simulink model "Project3_Part2_sim"  (R2018a)
(part 3 of 4)

CFG = [t1033+t1034+t1035+t1036+t1037+t1038+t1040+t1041+thDot1.*3.0-t433.*(t2.*3.99066170156947e-3+t251)+t202.*(t213+t241+t245+t250+t259+t271+t272+t276+t277+t281+t283+t287+t291+t292+t293+t294+t295+t296+t297+t298+t299+t300+t301+t302+t303+t304+t305+t306+t307+t308+t402+t405+t406+t407+t408+t442+t446-t2.*t14.*1.25890039900759e-2-t62.*t133.*1.139953928995173-t14.*t253.*7.377352061241174e1-t404.*thDot1.*4.38483060303202-t131.*(t183+t184+t186+t222-t8.*t27.*t109).*1.994855465224146-t2.*t12.*t14.*9.450145625450081e-1-t2.*t12.*t84.*9.450145625450081e-1-t2.*t12.*t86.*9.450145625450081e-1-t2.*t27.*t266.*4.38483060303202-t2.*t3.*t7.*t14.*1.865719029901695e-3-t2.*t3.*t7.*t84.*1.865719029901695e-3-t2.*t3.*t7.*t86.*1.865719029901695e-3-t2.*t3.*t7.*t87.*1.865719029901695e-3-t2.*t14.*t89.*t90.*1.547905453732908-t2.*t84.*t89.*t90.*1.547905453732908-t2.*t86.*t89.*t90.*1.547905453732908-t12.*t27.*t113.*thDot4.*1.900321864457165e1-t2.*t12.*thDot2.*thDot3.*1.890029125090016-t8.*t182.*thDot1.*thDot2.*3.812773007925995e1-t2.*t3.*t7.*thDot2.*thDot3.*3.73143805980339e-3-t4.*t7.*t8.*thDot1.*thDot4.*3.73143805980339e-3-t3.*t8.*t12.*thDot1.*thDot2.*3.73143805980339e-3-t3.*t8.*t12.*thDot1.*thDot3.*3.73143805980339e-3-t2.*t89.*t90.*thDot2.*thDot3.*3.095810907465815)+t33.*(t836+t33.*(t827+t828-t2.*t8.*t92.*2.36837910197578e-2)-t109.*t831)-t742.*(t213+t241+t245+t250+t259+t271+t272+t276+t277+t281+t283+t287+t291+t292+t293+t294+t295+t296+t297+t298+t299+t300+t301+t302+t303+t304+t305+t306+t307+t308+t507+t508+t509+t510-t2.*t14.*4.310799465649219e-3-t62.*t133.*1.139953928995173-t131.*t314.*1.994855465224146-t2.*t12.*t14.*9.450145625450081e-1-t2.*t12.*t84.*9.450145625450081e-1-t2.*t12.*t86.*9.450145625450081e-1-t2.*t3.*t7.*t14.*1.865719029901695e-3-t2.*t3.*t7.*t84.*1.865719029901695e-3-t2.*t3.*t7.*t86.*1.865719029901695e-3-t2.*t3.*t7.*t87.*1.865719029901695e-3-t2.*t14.*t89.*t90.*1.547905453732908-t2.*t84.*t89.*t90.*1.547905453732908-t2.*t86.*t89.*t90.*1.547905453732908-t12.*t27.*t113.*thDot4.*1.900321864457165e1-t2.*t12.*thDot2.*thDot3.*1.890029125090016-t2.*t3.*t7.*thDot2.*thDot3.*3.73143805980339e-3-t4.*t7.*t8.*thDot1.*thDot4.*3.73143805980339e-3-t3.*t8.*t12.*thDot1.*thDot2.*3.73143805980339e-3-t3.*t8.*t12.*thDot1.*thDot3.*3.73143805980339e-3-t2.*t89.*t90.*thDot2.*thDot3.*3.095810907465815)+t959.*(t340+t342+t347+t348+t349+t363+t364+t365+t366+t367+t368+t369+t370+t371+t372+t373+t377+t378+t379+t380+t563+t564+t565+t566+t567+t568+t569+t570+t571+t572+t573-t71.*t123.*1.139953928995173-t145.*t152.*1.139953928995173-t104.*t221.*1.994855465224146-t36.*t339.*1.994855465224146-t36.*t352.*1.139953928995173-t131.*t394.*1.994855465224146-t8.*t14.*t85.*8.455164471901305e-1-t8.*t84.*t85.*8.455164471901305e-1-t8.*t14.*t85.*t88.*2.191879307959464e-1-t8.*t84.*t85.*t88.*2.191879307959464e-1-t8.*t85.*t86.*t88.*2.191879307959464e-1-t2.*t4.*t7.*thDot1.*thDot4.*3.73143805980339e-3-t2.*t3.*t12.*thDot1.*thDot2.*3.73143805980339e-3-t2.*t3.*t12.*thDot1.*thDot3.*3.73143805980339e-3-t4.*t8.*t12.*thDot2.*thDot4.*3.73143805980339e-3-t4.*t8.*t12.*thDot3.*thDot4.*3.73143805980339e-3-t3.*t8.*t91.*thDot1.*thDot4.*3.73143805980339e-3-t3.*t8.*t92.*thDot1.*thDot4.*3.73143805980339e-3-t8.*t85.*t88.*thDot2.*thDot3.*4.383758615918928e-1)+t230.*(t340+t342+t347+t348+t349+t363+t364+t365+t366+t367+t368+t369+t370+t371+t372+t373+t374+t375+t376+t377+t378+t379+t380+t381+t382+t383+t384+t385+t386+t391+t398+t399+t400+t401-t434-t435-t436+t485-t486-t487-t488-t489-t490-t491-t492-t493-t494-t495-t496-t497-t498-t499-t500-t501-t502-t503-t504)+t172.*t438-t71.*t553-t226.*t433-t167.*t506-t140.*t597-t179.*t676-t134.*t730-t108.*t877-t107.*t890-t113.*t887-t290.*t711-t62.*t955-t314.*t733-t114.*t964-t397.*t713+t438.*t746+t553.*t901-t941.*(t340+t342+t347+t348+t349+t363+t364+t365+t366+t367+t368+t369+t370+t371+t372+t373+t374+t375+t376+t377+t378+t379+t380+t381+t382+t383+t384+t385+t398+t518+t519+t520-t71.*t123.*1.139953928995173-t33.*t211.*1.900321864457165e1-t145.*t152.*1.139953928995173-t104.*t221.*1.994855465224146-t36.*t339.*1.994855465224146-t36.*t352.*1.139953928995173-t109.*t344.*1.900321864457165e1-t131.*t394.*1.994855465224146-t8.*t14.*t85.*5.971038255043736-t8.*t84.*t85.*5.971038255043736-t8.*t14.*t85.*t88.*1.547905453732908-t8.*t84.*t85.*t88.*1.547905453732908-t8.*t85.*t86.*t88.*1.547905453732908-t12.*t27.*t179.*thDot4.*1.900321864457165e1-t2.*t4.*t7.*thDot1.*thDot4.*3.73143805980339e-3-t2.*t3.*t12.*thDot1.*thDot2.*3.73143805980339e-3-t2.*t3.*t12.*thDot1.*thDot3.*3.73143805980339e-3-t4.*t8.*t12.*thDot2.*thDot4.*3.73143805980339e-3-t4.*t8.*t12.*thDot3.*thDot4.*3.73143805980339e-3-t3.*t8.*t91.*thDot1.*thDot4.*3.73143805980339e-3-t3.*t8.*t92.*thDot1.*thDot4.*3.73143805980339e-3-t8.*t85.*t88.*thDot2.*thDot3.*3.095810907465815)-t7.*thDot4.*(1.0./1.0e1)-t64.*thDot6.*(1.0./2.0e1)-t506.*(t8.*3.99066170156947e-3-t201)+t683.*(t213+t241+t245+t250+t259+t464+t465+t466+t467+t468+t469+t470+t471+t472+t473+t474+t475+t476+t477+t478+t479+t480+t481+t482+t483+t484+t156.*(t21+t22+t23-t12.*thDot2.*thDot4-t12.*thDot3.*thDot4).*1.139953928995173-t2.*t14.*2.219760847427988e-4-t62.*t133.*1.139953928995173+t78.*(t183+t184+t185+t186-t36.*(t28+t32+t42-t2.*t12.*thDot4)+(thDot1-t7.*thDot4).*(t28+t32-t2.*t12.*thDot4)+t8.*t27.*(t34-thDot1)).*1.139953928995173-t2.*t12.*t14.*3.436486650567527e-1-t2.*t12.*t84.*3.436486650567527e-1-t2.*t12.*t86.*3.436486650567527e-1-t2.*t3.*t7.*t14.*6.784571152745185e-4-t2.*t3.*t7.*t84.*6.784571152745185e-4-t2.*t3.*t7.*t86.*6.784571152745185e-4-t2.*t3.*t7.*t87.*6.784571152745185e-4-t2.*t14.*t89.*t90.*7.970632707682899e-2-t2.*t84.*t89.*t90.*7.970632707682899e-2-t2.*t86.*t89.*t90.*7.970632707682899e-2-t2.*t12.*thDot2.*thDot3.*6.872973301135055e-1-t2.*t3.*t7.*thDot2.*thDot3.*1.356914230549037e-3-t4.*t7.*t8.*thDot1.*thDot4.*1.356914230549037e-3-t3.*t8.*t12.*thDot1.*thDot2.*1.356914230549037e-3-t3.*t8.*t12.*thDot1.*thDot3.*1.356914230549037e-3-t2.*t89.*t90.*thDot2.*thDot3.*1.59412654153658e-1)+t840.*(t213+t241+t245+t250+t259+t271+t276+t277+t283+t287+t292+t293+t297+t298+t299+t300+t301+t302+t303+t574+t575+t576+t577+t578+t579+t580+t581+t582+t583+t584+t585-t2.*t14.*6.104217881481557e-4-t62.*t133.*1.139953928995173-t131.*t314.*1.994855465224146-t2.*t12.*t14.*9.450145625450081e-1-t2.*t12.*t84.*9.450145625450081e-1-t2.*t12.*t86.*9.450145625450081e-1-t2.*t3.*t7.*t14.*1.865719029901695e-3-t2.*t3.*t7.*t84.*1.865719029901695e-3-t2.*t3.*t7.*t86.*1.865719029901695e-3-t2.*t3.*t7.*t87.*1.865719029901695e-3-t2.*t14.*t89.*t90.*2.191879307959464e-1-t2.*t84.*t89.*t90.*2.191879307959464e-1-t2.*t86.*t89.*t90.*2.191879307959464e-1-t2.*t12.*thDot2.*thDot3.*1.890029125090016-t2.*t3.*t7.*thDot2.*thDot3.*3.73143805980339e-3-t4.*t7.*t8.*thDot1.*thDot4.*3.73143805980339e-3-t3.*t8.*t12.*thDot1.*thDot2.*3.73143805980339e-3-t3.*t8.*t12.*thDot1.*thDot3.*3.73143805980339e-3-t2.*t89.*t90.*thDot2.*thDot3.*4.383758615918928e-1)+t253.*(t340+t342+t347+t348+t349+t363+t364+t365+t366+t367+t368+t369+t370+t371+t372+t373+t374+t375+t376+t377+t378+t379+t380+t381+t382+t383+t384+t385+t386+t391+t399+t400+t401+t429-t71.*t123.*1.139953928995173+t14.*t202.*7.377352061241174e1-t33.*t211.*1.900321864457165e1-t145.*t152.*1.139953928995173-t104.*t221.*1.994855465224146-t36.*t339.*1.994855465224146-t36.*t352.*1.139953928995173-t109.*t344.*1.900321864457165e1-t432.*thDot1.*3.812773007925995e1-t131.*(t124+t125+t126+t127-t2.*t27.*t109).*1.994855465224146+t164.*(t125+t127-t2.*t27.*t109).*1.900321864457165e1-t8.*t14.*t85.*7.153708691033507-t8.*t84.*t85.*7.153708691033507-t8.*t270.*thDot2.*3.812773007925995e1-t8.*t14.*t85.*t88.*1.547905453732908-t8.*t84.*t85.*t88.*1.547905453732908-t8.*t85.*t86.*t88.*1.547905453732908-t12.*t27.*t179.*thDot4.*1.900321864457165e1-t2.*t182.*thDot1.*thDot2.*3.812773007925995e1-t2.*t4.*t7.*thDot1.*thDot4.*3.73143805980339e-3-t2.*t3.*t12.*thDot1.*thDot2.*3.73143805980339e-3-t2.*t3.*t12.*thDot1.*thDot3.*3.73143805980339e-3-t4.*t8.*t12.*thDot2.*thDot4.*3.73143805980339e-3-t4.*t8.*t12.*thDot3.*thDot4.*3.73143805980339e-3-t3.*t8.*t91.*thDot1.*thDot4.*3.73143805980339e-3-t3.*t8.*t92.*thDot1.*thDot4.*3.73143805980339e-3-t8.*t85.*t88.*thDot2.*thDot3.*3.095810907465815)-t945.*(t340+t342+t347+t348+t349+t363+t364+t365+t366+t367+t368+t369+t370+t371+t372+t373+t374+t375+t376+t377+t378+t379+t380+t381+t382+t383+t384+t385+t386+t391+t398+t399+t400+t401+t485-t71.*t123.*1.139953928995173-t33.*t211.*1.900321864457165e1-t145.*t152.*1.139953928995173-t104.*t221.*1.994855465224146-t36.*t339.*1.994855465224146-t36.*t352.*1.139953928995173-t109.*t344.*1.900321864457165e1-t131.*t394.*1.994855465224146-t8.*t14.*t85.*7.153708691033507-t8.*t84.*t85.*7.153708691033507-t8.*t14.*t85.*t88.*1.547905453732908-t8.*t84.*t85.*t88.*1.547905453732908-t8.*t85.*t86.*t88.*1.547905453732908-t12.*t27.*t179.*thDot4.*1.900321864457165e1-t2.*t4.*t7.*thDot1.*thDot4.*3.73143805980339e-3-t2.*t3.*t12.*thDot1.*thDot2.*3.73143805980339e-3-t2.*t3.*t12.*thDot1.*thDot3.*3.73143805980339e-3-t4.*t8.*t12.*thDot2.*thDot4.*3.73143805980339e-3-t4.*t8.*t12.*thDot3.*thDot4.*3.73143805980339e-3-t3.*t8.*t91.*thDot1.*thDot4.*3.73143805980339e-3-t3.*t8.*t92.*thDot1.*thDot4.*3.73143805980339e-3-t8.*t85.*t88.*thDot2.*thDot3.*3.095810907465815)+t8.*t27.*t852+t2.*t27.*t967-t4.*t12.*thDot5.*(1.0./1.0e1)-t8.*t691.*thDot2-t2.*t904.*thDot2+t7.*t12.*t27.*t586.*thDot1.*9.31865436135962e-4+t7.*t12.*t27.*t587.*thDot1.*9.31865436135962e-4-t85.*t89.*t586.*thDot1.*thDot2.*1.778633004674423e-1-t85.*t89.*t587.*thDot1.*thDot2.*1.778633004674423e-1;t8.*(t1006+t1008+t1013+t1014+t1015+t1016+t1019+t1020+t1021+t1022+t1023+t1026+t1028+t1029+t1030+t1031+t1032+t683.*(t618+t619+t620+t621+t622+t623+t625+t626+t627+t628+t629+t630+t631+t632+t633+t634+t635+t636+t637+t638+t639+t640+t641+t642+t643+t644+t645+t646+t647+t648+t649+t650+t651+t652+t653+t654+t655+t656+t657+t658+t659+t660+t661+t856-t71.*t231.*1.139953928995173-t73.*t244.*1.139953928995173-t50.*t337.*1.139953928995173-t62.*t602.*1.139953928995173-t84.*t89.*t90.*3.436486650567527e-1-t86.*t89.*t90.*3.436486650567527e-1-t3.*t84.*t85.*t90.*6.784571152745185e-4-t3.*t84.*t88.*t89.*6.784571152745185e-4-t3.*t85.*t86.*t90.*6.784571152745185e-4-t3.*t85.*t87.*t90.*6.784571152745185e-4-t3.*t86.*t88.*t89.*6.784571152745185e-4-t3.*t87.*t88.*t89.*6.784571152745185e-4-t13.*t84.*t89.*t90.*1.199966622536514e-4-t13.*t86.*t89.*t90.*1.199966622536514e-4-t13.*t89.*t90.*t607.*1.199966622536514e-4-t89.*t90.*thDot2.*thDot3.*6.872973301135055e-1-t3.*t85.*t88.*thDot2.*thDot4.*4.530050512289873e-4-t3.*t85.*t88.*thDot3.*thDot4.*4.530050512289873e-4-t3.*t85.*t90.*thDot2.*thDot3.*1.356914230549037e-3-t4.*t85.*t88.*thDot2.*thDot4.*1.356914230549037e-3-t4.*t85.*t88.*thDot3.*thDot4.*1.356914230549037e-3-t3.*t88.*t89.*thDot2.*thDot3.*1.356914230549037e-3-t13.*t89.*t90.*thDot2.*thDot3.*2.399933245073028e-4-t4.*t11.*t89.*t90.*thDot2.*thDot4.*2.399933245073028e-4-t4.*t11.*t89.*t90.*thDot3.*thDot4.*2.399933245073028e-4-t4.*t13.*t85.*t90.*thDot4.*thDot5.*2.399933245073028e-4-t3.*t13.*t89.*t90.*thDot2.*thDot5.*2.399933245073028e-4-t3.*t13.*t89.*t90.*thDot3.*thDot5.*2.399933245073028e-4-t4.*t13.*t88.*t89.*thDot4.*thDot5.*2.399933245073028e-4+1.11715485041527e1)-t78.*t553-t164.*t676-t113.*t744-t175.*t737-t123.*t855-t397.*t601-t108.*t910-t394.*t680-t109.*t1025-t337.*t821+t597.*t889-t742.*t744+t746.*t826-t737.*t920-t880.*t1012+t8.*thDot2.*3.0+t691.*thDot1-t852.*thDot1-t62.*(t946+t949-t62.*t799)+t182.*(t340+t347+t348+t349+t363+t364+t365+t366+t367+t368+t369+t370+t371+t372+t373+t374+t375+t376+t377+t378+t379+t380+t381+t382+t383+t384+t385+t386+t391+t398+t399+t400+t401+t429-t434-t435-t436-t486-t487-t488-t489-t490-t491-t492-t493-t494-t495-t496-t497-t498-t499-t500-t501-t502-t503-t504+t723-t738-t739-t740)-t107.*(t608+t611+t612+t616+t617+t618+t619+t620+t621+t622+t623+t624+t625+t626+t627+t628+t629+t630+t631+t632+t633+t634+t635+t636+t637+t638+t639+t640+t641+t642+t643+t644+t645+t646+t647+t648+t649+t650+t651+t652+t653+t654+t655+t656+t657+t658+t659+t660+t661+t662+t841+t842+t843+t844-t71.*t231.*1.139953928995173-t73.*t244.*1.139953928995173-t104.*t275.*1.994855465224146-t50.*t337.*1.139953928995173-t140.*t314.*1.994855465224146-t62.*t602.*1.139953928995173-t84.*t604.*5.936309573135882e-4-t84.*t606.*5.936309573135882e-4-t86.*t604.*5.936309573135882e-4-t87.*t604.*5.936309573135882e-4-t86.*t606.*5.936309573135882e-4-t87.*t606.*5.936309573135882e-4-t84.*t89.*t90.*3.436486650567527e-1-t86.*t89.*t90.*3.436486650567527e-1-t604.*thDot2.*thDot3.*1.187261914627176e-3-t604.*thDot2.*thDot4.*1.187261914627176e-3-t604.*thDot3.*thDot4.*1.187261914627176e-3-t606.*thDot2.*thDot3.*1.187261914627176e-3-t3.*t84.*t85.*t90.*6.784571152745185e-4-t3.*t84.*t88.*t89.*6.784571152745185e-4-t3.*t85.*t86.*t90.*6.784571152745185e-4-t3.*t85.*t87.*t90.*6.784571152745185e-4-t3.*t86.*t88.*t89.*6.784571152745185e-4-t3.*t87.*t88.*t89.*6.784571152745185e-4-t13.*t84.*t89.*t90.*1.199966622536514e-4-t13.*t86.*t89.*t90.*1.199966622536514e-4-t13.*t89.*t90.*t607.*1.199966622536514e-4-t89.*t90.*thDot2.*thDot3.*6.872973301135055e-1-t3.*t85.*t88.*thDot2.*thDot4.*4.530050512289873e-4-t3.*t85.*t88.*thDot3.*thDot4.*4.530050512289873e-4-t3.*t85.*t90.*thDot2.*thDot3.*1.356914230549037e-3-t4.*t85.*t88.*thDot2.*thDot4.*1.356914230549037e-3-t4.*t85.*t88.*thDot3.*thDot4.*1.356914230549037e-3-t3.*t88.*t89.*thDot2.*thDot3.*1.356914230549037e-3-t13.*t89.*t90.*thDot2.*thDot3.*2.399933245073028e-4-t4.*t11.*t89.*t90.*thDot2.*thDot4.*2.399933245073028e-4-t4.*t11.*t89.*t90.*thDot3.*thDot4.*2.399933245073028e-4-t4.*t13.*t85.*t90.*thDot4.*thDot5.*2.399933245073028e-4-t3.*t13.*t89.*t90.*thDot2.*thDot5.*2.399933245073028e-4-t3.*t13.*t89.*t90.*thDot3.*thDot5.*2.399933245073028e-4-t4.*t13.*t88.*t89.*thDot4.*thDot5.*2.399933245073028e-4+3.072113206334932e1)-t167.*(t608+t609+t610+t611+t612+t613+t614+t615+t616+t617+t618+t619+t620+t621+t622+t623+t624+t625+t626+t627+t628+t629+t630+t631+t632+t633+t634+t635+t636+t637+t638+t639+t640+t641+t642+t643+t644+t645+t646+t647+t648+t649+t650+t651+t652+t653+t654+t655+t656+t657+t658+t659+t660+t661+t662+t748+t764+t770+t884+t885-t71.*t231.*1.139953928995173-t73.*t244.*1.139953928995173-t104.*t275.*1.994855465224146-t50.*t337.*1.139953928995173-t140.*t314.*1.994855465224146-t114.*t344.*1.900321864457165e1-t179.*t290.*1.900321864457165e1-t62.*t602.*1.139953928995173-t84.*t604.*5.936309573135882e-4-t84.*t606.*5.936309573135882e-4-t86.*t604.*5.936309573135882e-4-t87.*t604.*5.936309573135882e-4-t86.*t606.*5.936309573135882e-4-t87.*t606.*5.936309573135882e-4-t84.*t89.*t90.*3.436486650567527e-1-t86.*t89.*t90.*3.436486650567527e-1-t8.*t27.*t404.*4.38483060303202-t2.*t432.*thDot2.*3.812773007925995e1-t604.*thDot2.*thDot3.*1.187261914627176e-3-t604.*thDot2.*thDot4.*1.187261914627176e-3-t604.*thDot3.*thDot4.*1.187261914627176e-3-t606.*thDot2.*thDot3.*1.187261914627176e-3-t3.*t84.*t85.*t90.*6.784571152745185e-4-t3.*t84.*t88.*t89.*6.784571152745185e-4-t3.*t85.*t86.*t90.*6.784571152745185e-4-t3.*t85.*t87.*t90.*6.784571152745185e-4-t3.*t86.*t88.*t89.*6.784571152745185e-4-t3.*t87.*t88.*t89.*6.784571152745185e-4-t13.*t84.*t89.*t90.*1.199966622536514e-4-t13.*t86.*t89.*t90.*1.199966622536514e-4-t13.*t89.*t90.*t607.*1.199966622536514e-4-t2.*t27.*t172.*thDot1.*4.38483060303202-t89.*t90.*thDot2.*thDot3.*6.872973301135055e-1-t8.*t226.*thDot1.*thDot2.*3.812773007925995e1-t3.*t85.*t88.*thDot2.*thDot4.*4.530050512289873e-4-t3.*t85.*t88.*thDot3.*thDot4.*4.530050512289873e-4-t3.*t85.*t90.*thDot2.*thDot3.*1.356914230549037e-3-t4.*t85.*t88.*thDot2.*thDot4.*1.356914230549037e-3-t4.*t85.*t88.*thDot3.*thDot4.*1.356914230549037e-3-t3.*t88.*t89.*thDot2.*thDot3.*1.356914230549037e-3-t13.*t89.*t90.*thDot2.*thDot3.*2.399933245073028e-4-t4.*t11.*t89.*t90.*thDot2.*thDot4.*2.399933245073028e-4-t4.*t11.*t89.*t90.*thDot3.*thDot4.*2.399933245073028e-4-t4.*t13.*t85.*t90.*thDot4.*thDot5.*2.399933245073028e-4-t3.*t13.*t89.*t90.*thDot2.*thDot5.*2.399933245073028e-4-t3.*t13.*t89.*t90.*thDot3.*thDot5.*2.399933245073028e-4-t4.*t13.*t88.*t89.*thDot4.*thDot5.*2.399933245073028e-4+6.335757694666128e2)-t2.*t12.*thDot4.*(1.0./1.0e1)-t8.*t27.*t595.*thDot1-t2.*t27.*t868.*thDot1-t8.*t592.*thDot1.*thDot2-t2.*t872.*thDot1.*thDot2+t2.*t977.*thDot1.*thDot2)+t2.*(t979+t980+t981+t983+t985+t986+t987+t988+t989+t990+t992+t993+t994+t995+t996+t998+t999+t1000+t1002+t1003+t1004-t182.*t506-t36.*t877-t33.*t896-t71.*t882-t337.*t673-t66.*t955-t131.*t890-t140.*t891-t179.*t942-t394.*t806-t397.*t912+t438.*t920-t826.*t945-t889.*t890-t887.*t969-t941.*t942+t2.*thDot2.*3.0+t904.*thDot1-t967.*thDot1-t226.*(t608+t609+t610+t611+t612+t613+t614+t615+t616+t617+t618+t619+t620+t621+t622+t623+t624+t625+t626+t627+t628+t629+t630+t631+t632+t633+t634+t635+t636+t637+t638+t639+t640+t641+t642+t643+t644+t645+t646+t647+t648+t649+t650+t651+t652+t653+t654+t655+t656+t657+t658+t659+t660+t661-t747+t748-t749-t750-t751-t752-t753-t754-t755-t756-t757-t758-t759-t760-t761-t762-t763+t764-t765-t766-t767-t768-t769+t770-t771-t772-t773-t774-t775-t776-t777-t778-t779-t780-t781-t782-t783-t784-t785-t786-t787-t788-t789-t790-t791-t792+t825-t883+t884+t885-t886-t2.*t432.*thDot2.*3.812773007925995e1-t8.*t226.*thDot1.*thDot2.*3.812773007925995e1+6.335757694666128e2)-t12.*t27.*t831.*thDot4-t8.*t27.*t973.*thDot1+t2.*t592.*thDot1.*thDot2+t8.*t687.*thDot1.*thDot2-t8.*t977.*thDot1.*thDot2);t8.*(t1006+t1008+t1013+t1014+t1015+t1016+t1019+t1020+t1021+t1022+t1023+t1026+t1028+t1029+t1030+t1031+t1032+t1042+t1043-t175.*t737-t123.*t855-t107.*t891-t397.*t601-t108.*t910-t113.*t942-t394.*t680-t62.*t1018-t78.*t1012-t109.*t1025-t337.*t821-t164.*t1009-t742.*t942-t880.*t1012-t852.*thDot1-t2.*t12.*thDot4.*(1.0./1.0e1)-t8.*t27.*t595.*thDot1-t2.*t27.*t868.*thDot1)+t2.*(t979+t980+t981+t983+t985+t986+t987+t988+t989+t990+t992+t993+t994+t995+t996+t998+t999+t1000+t1002+t1003+t1004-t36.*t877-t33.*t896-t71.*t882-t337.*t673-t66.*t955-t131.*t890-t140.*t891-t179.*t942-t394.*t806-t397.*t912-t889.*t890-t887.*t969-t941.*t942-t967.*thDot1-t12.*t27.*t831.*thDot4-t8.*t27.*t973.*thDot1);t7.*(-t1033-t1034-t1035-t1036-t1037-t1038-t1040-t1041+t1050+t1051+t1052+t1053+t1054+t1055+t1056+t1057+t1058+t113.*t887+t290.*t711-t33.*t1025+t114.*t964+t397.*t713+t179.*t1009-t683.*t881-t840.*t890-t901.*t1012-t959.*t1005+t7.*thDot4.*(1.0./1.0e1))+t8.*t12.*(t979+t980+t981+t983+t985+t986+t988+t989+t990+t993+t995+t996+t998+t999+t1002+t1049-t36.*t877-t33.*t896-t71.*t882-t337.*t673-t131.*t890-t140.*t891-t66.*t1048-t179.*t942-t394.*t806-t397.*t912-t889.*t890-t12.*t27.*t831.*thDot4)-t2.*t12.*(t1006+t1008+t1013+t1014+t1015+t1016+t1019+t1020+t1022+t1026+t1028+t1029+t1032+t1042+t1043-t123.*t855-t107.*t891-t397.*t601-t108.*t910-t113.*t942-t394.*t680-t62.*t1018-t78.*t1012-t109.*t1025-t164.*t1009-t337.*t1045-t880.*t1012-t2.*t12.*thDot4.*(1.0./1.0e1));t17.*(t979+t980+t983+t985+t986+t988+t989+t990+t993+t995+t1049-t36.*t877-t71.*t882-t337.*t673-t131.*t890-t140.*t891-t66.*t1048-t394.*t806)+t31.*(t1006+t1008+t1015+t1016+t1019+t1020+t1022+t1028+t1029+t1043-t123.*t855-t107.*t891-t108.*t910-t394.*t680-t62.*t1018-t78.*t1012-t337.*t1045-t880.*t1012)-t4.*t12.*(t1033+t1034+t1035+t1036+t1037+t1038+t1040-t1050-t1051-t1052-t1053-t1054-t1055-t1056-t1057-t1058+t683.*t881+t901.*t1012);t41.*(t1008+t1016+t1019+t1028-t123.*t855-t62.*t1018-t78.*t1012-t337.*t1045)+t58.*(t983+t988+t989+t992+t993-t71.*t882-t337.*t673-t66.*t1048)-t64.*(t1033+t1034+t1035+t1037+t1038-t1053-t1054-t1055)];
end
